simulink model "px4demo_HostSerial_TxRx"  (R2017b)
settings: Solver=VariableStepAuto  StartTime=0.0  StopTime=inf  RelTol=1e-3  EnableMultiTasking=on
undefined symbols (not defined in the file or in its folder): serial
libraries: instrumentlib x3, aerolibanimutils x1
Description:
  | PX4 PSP Demo Showing Host side Serial communication
  | 
  | Host-side Serial Rx / Tx
settings Model: Creator=darenlee  LastModifiedBy=skuznick
settings DataIOCC: LimitDataPoints=on
settings OptimizationCC: LifeSpan=inf
settings DebuggingCC: AllowSymbolicDim=off  SFUnexpectedBacktrackingDiag=warning  SFNoUnconditionalDefaultTransitionDiag=warning  SFExecutionAtInitializationDiag=none
settings ModelReferenceCC: PropagateSignalLabelsOutOfModel=off
settings CodeAppCC: StateflowObjectComments=on
settings GRTTargetCC: TargetLangStandard=C89/C90 (ANSI)
settings ConfigComp: CovMetricSettings=dw  CovHtmlReporting=on  CovSaveCumulativeToWorkspaceVar=on  CovSaveSingleToWorkspaceVar=on  CovExternalEMLEnable=off

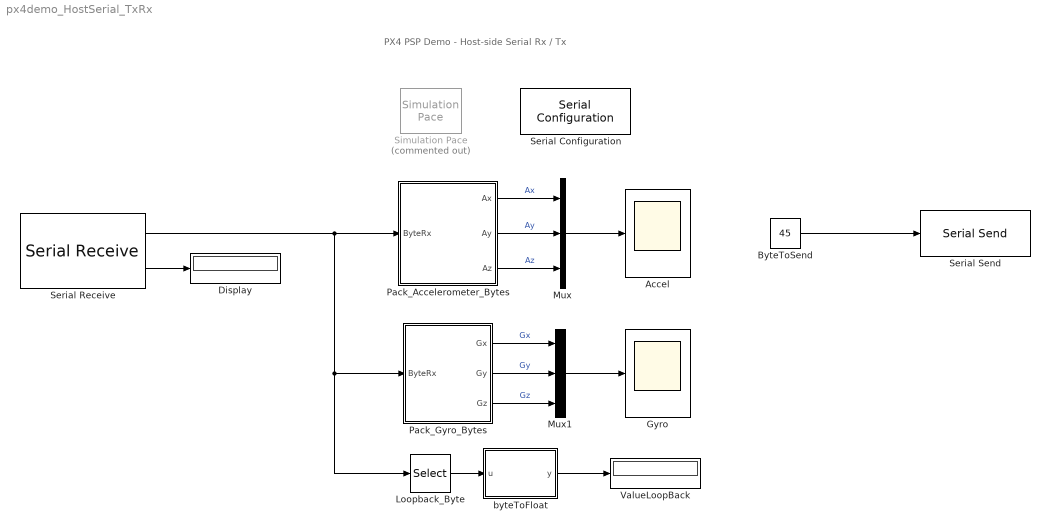
== system px4demo_HostSerial_TxRx ==
  note: PX4 PSP Demo - Host-side Serial Rx / Tx
  Accel : Scope
  ByteToSend : Constant  Value=45  OutDataTypeStr=uint8  SampleTime=0.005
  Display : Display
  Gyro : Scope
  Loopback_Byte : Selector  InputPortWidth=28  IndexOptions=Index vector (dialog)  Indices=25:28  OutputSizes=1
  Mux : Mux  Inputs=3
  Mux1 : Mux  Inputs=3
  Pack_Accelerometer_Bytes : Subsystem
  Pack_Gyro_Bytes : Subsystem
  Serial Configuration : instrumentlib/Serial Configuration  Priority=-200000  ComPortMenu=<Please select a port...>  ComPort=COM6  ObjConstructor=serial('COM6');  BaudRate=115200  DataBits=8  Parity=none  StopBits=1  FlowControl=none  Timeout=10  ByteOrder=LittleEndian
  Serial Receive : instrumentlib/Serial Receive  ComPortMenu=<Please select a port...>  ComPort=COM6  ObjConstructor=serial('COM6');  Terminator=<none>  DataSize="[28   1]"  DataType=uint8  EnableBlockingMode=off  ActionDataUnavailable=Output last received value  CustomValue=0  SampleTime=0.005
  Serial Send : instrumentlib/Serial Send  ComPortMenu=<Please select a port...>  ComPort=COM6  ObjConstructor=serial('COM6');  Terminator=<none>  EnableBlockingMode=off
  Simulation Pace : aerolibanimutils/Simulation Pace  Commented=on  SimulationPace=1  SleepMode=MATLAB Thread  OutputPaceError=off  SampleTime=0.005
  ValueLoopBack : Display
  byteToFloat : MATLAB Function  TreatAsAtomicUnit=on
  wires:
  Mux/1 -> Accel/1
  Pack_Accelerometer_Bytes/2(Ay) -> Mux/2  "Ay"
  Pack_Accelerometer_Bytes/1(Ax) -> Mux/1  "Ax"
  Pack_Accelerometer_Bytes/3(Az) -> Mux/3  "Az"
  Serial Receive/1 -> Pack_Accelerometer_Bytes/1(ByteRx), Loopback_Byte/1, Pack_Gyro_Bytes/1(ByteRx)
  Mux1/1 -> Gyro/1
  Pack_Gyro_Bytes/2(Gy) -> Mux1/2  "Gy"
  Pack_Gyro_Bytes/1(Gx) -> Mux1/1  "Gx"
  Pack_Gyro_Bytes/3(Gz) -> Mux1/3  "Gz"
  Loopback_Byte/1 -> byteToFloat/1(u)
  byteToFloat/1(y) -> ValueLoopBack/1
  ByteToSend/1 -> Serial Send/1
  Serial Receive/2 -> Display/1

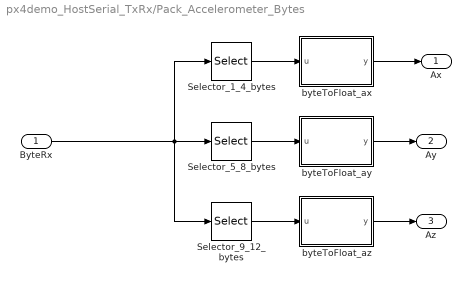
== system px4demo_HostSerial_TxRx/Pack_Accelerometer_Bytes ==
  ByteRx : Inport
  Selector_1_4_bytes : Selector  InputPortWidth=28  IndexOptions=Index vector (dialog)  Indices=[1:4]  OutputSizes=1
  Selector_5_8_bytes : Selector  InputPortWidth=28  IndexOptions=Index vector (dialog)  Indices=[5 6 7 8]  OutputSizes=1
  Selector_9_12_bytes : Selector  InputPortWidth=28  IndexOptions=Index vector (dialog)  Indices=[9 10 11 12]  OutputSizes=1
  byteToFloat_ax : MATLAB Function  TreatAsAtomicUnit=on
  byteToFloat_ay : MATLAB Function  TreatAsAtomicUnit=on
  byteToFloat_az : MATLAB Function  TreatAsAtomicUnit=on
  Ax : Outport
  Ay : Outport  Port=2
  Az : Outport  Port=3
  wires:
  byteToFloat_az/1(y) -> Az/1
  ByteRx/1 -> Selector_9_12_bytes/1, Selector_1_4_bytes/1, Selector_5_8_bytes/1
  byteToFloat_ax/1(y) -> Ax/1
  Selector_1_4_bytes/1 -> byteToFloat_ax/1(u)
  Selector_9_12_bytes/1 -> byteToFloat_az/1(u)
  Selector_5_8_bytes/1 -> byteToFloat_ay/1(u)
  byteToFloat_ay/1(y) -> Ay/1

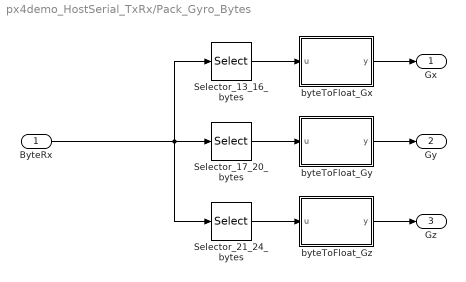
== system px4demo_HostSerial_TxRx/Pack_Gyro_Bytes ==
  ByteRx : Inport
  Selector_13_16_bytes : Selector  InputPortWidth=28  IndexOptions=Index vector (dialog)  Indices=[13 14 15 16]  OutputSizes=1
  Selector_17_20_bytes : Selector  InputPortWidth=28  IndexOptions=Index vector (dialog)  Indices=[17:20]  OutputSizes=1
  Selector_21_24_bytes : Selector  InputPortWidth=28  IndexOptions=Index vector (dialog)  Indices=[21:24]  OutputSizes=1
  byteToFloat_Gx : MATLAB Function  TreatAsAtomicUnit=on
  byteToFloat_Gy : MATLAB Function  TreatAsAtomicUnit=on
  byteToFloat_Gz : MATLAB Function  TreatAsAtomicUnit=on
  Gx : Outport
  Gy : Outport  Port=2
  Gz : Outport  Port=3
  wires:
  byteToFloat_Gz/1(y) -> Gz/1
  ByteRx/1 -> Selector_21_24_bytes/1, Selector_17_20_bytes/1, Selector_13_16_bytes/1
  byteToFloat_Gx/1(y) -> Gx/1
  Selector_13_16_bytes/1 -> byteToFloat_Gx/1(u)
  Selector_21_24_bytes/1 -> byteToFloat_Gz/1(u)
  Selector_17_20_bytes/1 -> byteToFloat_Gy/1(u)
  byteToFloat_Gy/1(y) -> Gy/1

== matlab function px4demo_HostSerial_TxRx/Pack_Accelerometer_Bytes/byteToFloat_ay ==
  data: u input; y output
function y = fcn(u)
%#codegen
y = single(0);
y = single(typecast(uint8(u),'single'));
% y = u;

== matlab function px4demo_HostSerial_TxRx/Pack_Accelerometer_Bytes/byteToFloat_ax ==
  data: u input; y output
function y = fcn(u)
%#codegen
y = single(0);
y = single(typecast(uint8(u),'single'));
% y = u;

== matlab function px4demo_HostSerial_TxRx/Pack_Accelerometer_Bytes/byteToFloat_az ==
  data: u input; y output
function y = fcn(u)
%#codegen
y = single(0);
y = single(typecast(uint8(u),'single'));
% y = u;

== matlab function px4demo_HostSerial_TxRx/Pack_Gyro_Bytes/byteToFloat_Gx ==
  data: u input; y output
function y = fcn(u)
%#codegen
y = single(0);
y = single(typecast(uint8(u),'single'));
% y = u;

== matlab function px4demo_HostSerial_TxRx/Pack_Gyro_Bytes/byteToFloat_Gy ==
  data: u input; y output
function y = fcn(u)
%#codegen
y = single(0);
y = single(typecast(uint8(u),'single'));
% y = u;

== matlab function px4demo_HostSerial_TxRx/Pack_Gyro_Bytes/byteToFloat_Gz ==
  data: u input; y output
function y = fcn(u)
%#codegen
y = single(0);
y = single(typecast(uint8(u),'single'));
% y = u;

== matlab function px4demo_HostSerial_TxRx/byteToFloat ==
  data: u input; y output
function y = fcn(u)
%#codegen
y = single(0);
y = single(typecast(uint8(u),'single'));
% y = u;
